simulink library "Ultrastick_Aero_Lib"  (Simulink 7.5)
settings: Solver=ode45  StartTime=0.0  StopTime=10.0  RelTol=1e-3
values from neighbouring files (symbols this model uses):
  AC = FASER_config    [UAV_config.m]    (also in UAV_modelconfig.mat = )
libraries: simulink x2
settings Model: Creator=austinmurch  LastModifiedBy=austinmurch

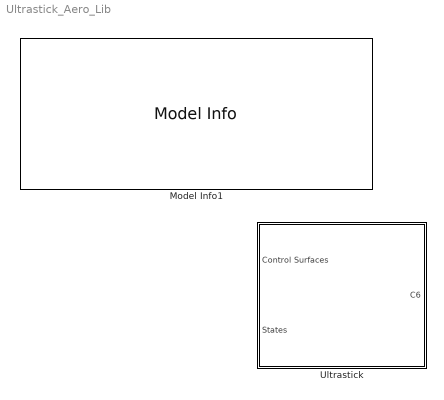
== system Ultrastick_Aero_Lib ==
  Model Info1 : simulink/Model-Wide Utilities/Model Info  SystemSampleTime=-1  InitialBlockCM=None  BlockCM=None  Frame=on  DisplayStringWithTags=|  HorizontalTextAlignment=Left  LeftAlignmentValue=0.02  SourceBlockDiagram=Ultrastick_Aero_Lib  TagMaxNumber=20
      | MODEL INFORMATION
      | Ultra Stick Aerodynamic Model Library
      | 
      | University of Minnesota
      | Aerospace Engineering and Mechanics
      | Copyright 2011 Regents of the University of Minnesota. All rights reserved.
      | 
      | == SVN Info ==
      | %<ModelVersion>
      | Last modified by %<LastModifiedBy> on %<LastModificationDate>
  Ultrastick : Subsystem

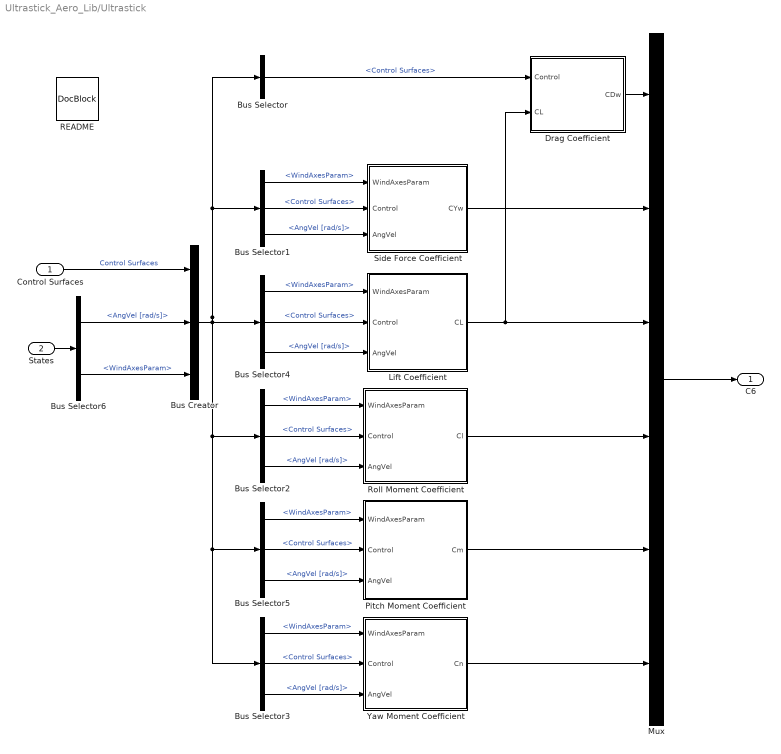
== system Ultrastick_Aero_Lib/Ultrastick ==
  Control Surfaces : Inport
  States : Inport  Port=2  OutDataType=sfix(16)  OutScaling=2^0
  Bus Creator : BusCreator  Inputs=3
  Bus Selector : BusSelector  OutputSignals=Control Surfaces
  Bus Selector{1..5} (5 alike) : BusSelector  OutputSignals=WindAxesParam,Control Surfaces,AngVel [rad/s]
  Bus Selector6 : BusSelector  OutputSignals=AngVel [rad/s],WindAxesParam
  Drag Coefficient : Subsystem
  Lift Coefficient : Subsystem
  Mux : Mux  Inputs=6
  Pitch Moment Coefficient : Subsystem
  README : simulink/Model-Wide Utilities/DocBlock  SystemSampleTime=-1  DocumentType=Text
  Roll Moment Coefficient : Subsystem
  Side Force Coefficient : Subsystem
  Yaw Moment Coefficient : Subsystem
  C6 : Outport  OutDataType=sfix(16)  OutScaling=2^0
  wires:
  Bus Selector/1 -> Drag Coefficient/1(Control)  "<Control Surfaces>"
  Control Surfaces/1 -> Bus Creator/1  "Control Surfaces"
  Bus Selector5/3 -> Pitch Moment Coefficient/3(AngVel)  "<AngVel [rad/s]>"
  Bus Selector5/2 -> Pitch Moment Coefficient/2(Control)  "<Control Surfaces>"
  Bus Selector5/1 -> Pitch Moment Coefficient/1(WindAxesParam)  "<WindAxesParam>"
  Bus Selector4/3 -> Lift Coefficient/3(AngVel)  "<AngVel [rad/s]>"
  Bus Selector4/2 -> Lift Coefficient/2(Control)  "<Control Surfaces>"
  Bus Selector4/1 -> Lift Coefficient/1(WindAxesParam)  "<WindAxesParam>"
  Bus Selector3/3 -> Yaw Moment Coefficient/3(AngVel)  "<AngVel [rad/s]>"
  Bus Selector3/2 -> Yaw Moment Coefficient/2(Control)  "<Control Surfaces>"
  Bus Selector3/1 -> Yaw Moment Coefficient/1(WindAxesParam)  "<WindAxesParam>"
  Bus Selector2/3 -> Roll Moment Coefficient/3(AngVel)  "<AngVel [rad/s]>"
  Bus Selector2/2 -> Roll Moment Coefficient/2(Control)  "<Control Surfaces>"
  Bus Selector2/1 -> Roll Moment Coefficient/1(WindAxesParam)  "<WindAxesParam>"
  Bus Selector1/3 -> Side Force Coefficient/3(AngVel)  "<AngVel [rad/s]>"
  Bus Selector1/2 -> Side Force Coefficient/2(Control)  "<Control Surfaces>"
  Bus Selector1/1 -> Side Force Coefficient/1(WindAxesParam)  "<WindAxesParam>"
  Bus Creator/1 -> Bus Selector4/1, Bus Selector1/1, Bus Selector/1, Bus Selector5/1, Bus Selector3/1, Bus Selector2/1
  Mux/1 -> C6/1
  Yaw Moment Coefficient/1(Cn) -> Mux/6
  Pitch Moment Coefficient/1(Cm) -> Mux/5
  Roll Moment Coefficient/1(Cl) -> Mux/4
  Side Force Coefficient/1(CYw) -> Mux/2
  Drag Coefficient/1(CDw) -> Mux/1
  States/1 -> Bus Selector6/1
  Bus Selector6/1 -> Bus Creator/2  "<AngVel [rad/s]>"
  Bus Selector6/2 -> Bus Creator/3  "<WindAxesParam>"
  Lift Coefficient/1(CL) -> Mux/3, Drag Coefficient/2(CL)

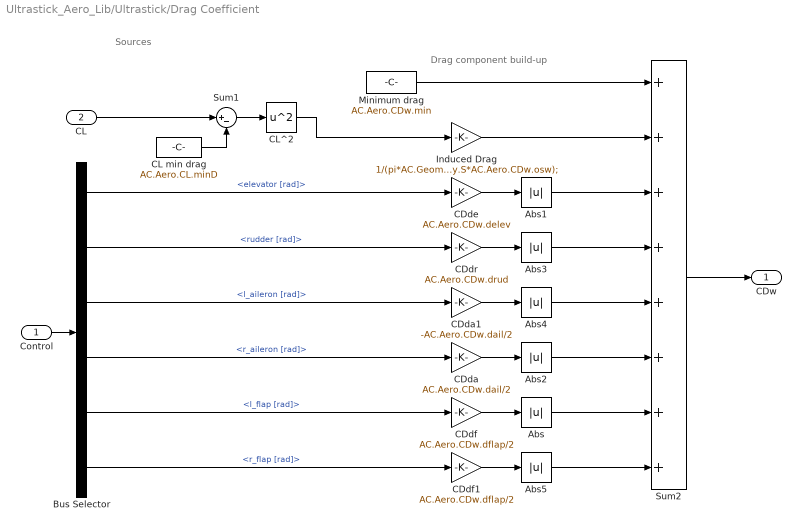
== system Ultrastick_Aero_Lib/Ultrastick/Drag Coefficient ==
  note: Drag component build-up
  note: Sources
  Control : Inport  OutDataType=sfix(16)  OutScaling=2^0
  CL : Inport  Port=2  OutDataType=sfix(16)  OutScaling=2^0
  Abs{,1..5} (6 alike) : Abs  SaturateOnIntegerOverflow=on
  Bus Selector : BusSelector  OutputSignals=elevator [rad],rudder [rad],l_aileron [rad],r_aileron [rad],l_flap [rad],r_flap [rad]
  CDda : Gain  Gain=AC.Aero.CDw.dail/2  ParameterDataType=sfix(16)  ParameterScaling=2^0  OutDataType=sfix(16)  OutScaling=2^0  SaturateOnIntegerOverflow=on  OutDataTypeStr=Inherit: Same as input  ParamDataTypeStr=Inherit: Same as input
  CDda1 : Gain  Gain=-AC.Aero.CDw.dail/2  ParameterDataType=sfix(16)  ParameterScaling=2^0  OutDataType=sfix(16)  OutScaling=2^0  SaturateOnIntegerOverflow=on  OutDataTypeStr=Inherit: Same as input  ParamDataTypeStr=Inherit: Same as input
  CDde : Gain  Gain=AC.Aero.CDw.delev  ParameterDataType=sfix(16)  ParameterScaling=2^0  OutDataType=sfix(16)  OutScaling=2^0  SaturateOnIntegerOverflow=on  OutDataTypeStr=Inherit: Same as input  ParamDataTypeStr=Inherit: Same as input
  CDdf : Gain  Gain=AC.Aero.CDw.dflap/2  ParameterDataType=sfix(16)  ParameterScaling=2^0  OutDataType=sfix(16)  OutScaling=2^0  SaturateOnIntegerOverflow=on  OutDataTypeStr=Inherit: Same as input  ParamDataTypeStr=Inherit: Same as input
  CDdf1 : Gain  Gain=AC.Aero.CDw.dflap/2  ParameterDataType=sfix(16)  ParameterScaling=2^0  OutDataType=sfix(16)  OutScaling=2^0  SaturateOnIntegerOverflow=on  OutDataTypeStr=Inherit: Same as input  ParamDataTypeStr=Inherit: Same as input
  CDdr : Gain  Gain=AC.Aero.CDw.drud  ParameterDataType=sfix(16)  ParameterScaling=2^0  OutDataType=sfix(16)  OutScaling=2^0  SaturateOnIntegerOverflow=on  OutDataTypeStr=Inherit: Same as input  ParamDataTypeStr=Inherit: Same as input
  CL min drag : Constant  Value=AC.Aero.CL.minD  OutDataType=sfix(16)  OutScaling=2^0
  CL^2 : Math  Operator=square  SaturateOnIntegerOverflow=on
  Induced Drag : Gain  Gain=1/(pi*AC.Geometry.b^2/AC.Geometry.S*AC.Aero.CDw.osw);  ParameterDataType=sfix(16)  ParameterScaling=2^0  OutDataType=sfix(16)  OutScaling=2^0  SaturateOnIntegerOverflow=on  OutDataTypeStr=Inherit: Same as input  ParamDataTypeStr=Inherit: Same as input
  Minimum drag : Constant  Value=AC.Aero.CDw.min  OutDataType=sfix(16)  OutScaling=2^0
  Sum1 : Sum  Inputs=|+-  OutDataType=sfix(16)  OutScaling=2^0  SaturateOnIntegerOverflow=on  InputSameDT=on  OutDataTypeStr=Inherit: Same as first input
  Sum2 : Sum  Inputs=++++++++  OutDataType=sfix(16)  OutScaling=2^0  SaturateOnIntegerOverflow=on  InputSameDT=on  OutDataTypeStr=Inherit: Same as first input
  CDw : Outport
  wires:
  Bus Selector/6 -> CDdf1/1  "<r_flap [rad]>"
  Abs/1 -> Sum2/7
  Abs5/1 -> Sum2/8
  CDdf1/1 -> Abs5/1
  Bus Selector/3 -> CDda1/1  "<l_aileron [rad]>"
  Abs4/1 -> Sum2/5
  CDda1/1 -> Abs4/1
  Abs2/1 -> Sum2/6
  Bus Selector/4 -> CDda/1  "<r_aileron [rad]>"
  Abs3/1 -> Sum2/4
  Abs1/1 -> Sum2/3
  CL min drag/1 -> Sum1/2
  CL/1 -> Sum1/1
  Sum1/1 -> CL^2/1
  Sum2/1 -> CDw/1
  CDdr/1 -> Abs3/1
  CDda/1 -> Abs2/1
  CDde/1 -> Abs1/1
  CDdf/1 -> Abs/1
  Induced Drag/1 -> Sum2/2
  Minimum drag/1 -> Sum2/1
  CL^2/1 -> Induced Drag/1
  Control/1 -> Bus Selector/1
  Bus Selector/2 -> CDdr/1  "<rudder [rad]>"
  Bus Selector/1 -> CDde/1  "<elevator [rad]>"
  Bus Selector/5 -> CDdf/1  "<l_flap [rad]>"

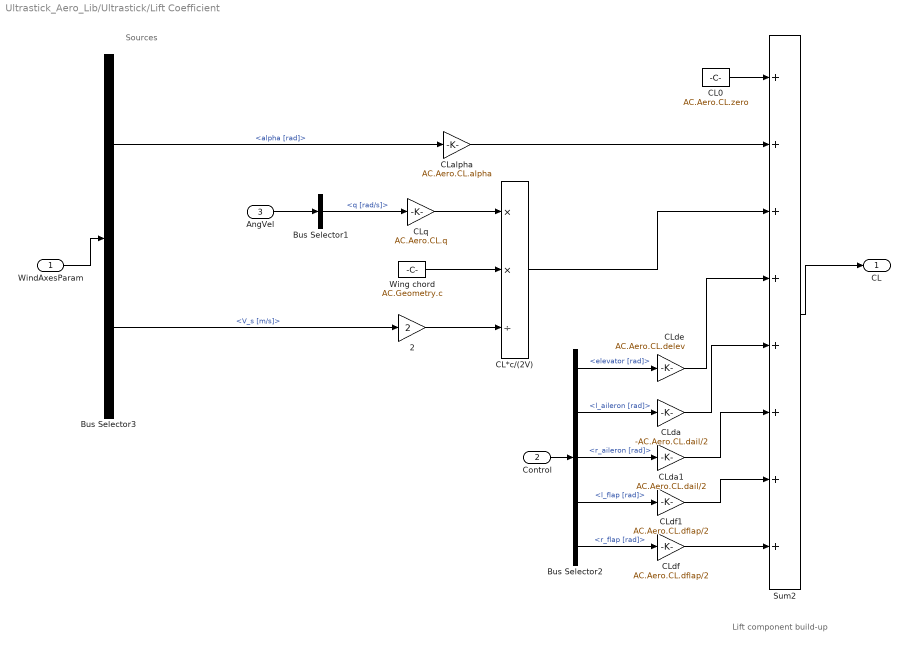
== system Ultrastick_Aero_Lib/Ultrastick/Lift Coefficient ==
  note: Lift component build-up
  note: Sources
  WindAxesParam : Inport  OutDataType=sfix(16)  OutScaling=2^0
  Control : Inport  Port=2  OutDataType=sfix(16)  OutScaling=2^0
  AngVel : Inport  Port=3  OutDataType=sfix(16)  OutScaling=2^0
  2 : Gain  Gain=2  ParameterDataType=sfix(16)  ParameterScaling=2^0  OutDataType=sfix(16)  OutScaling=2^0  SaturateOnIntegerOverflow=on  OutDataTypeStr=Inherit: Same as input  ParamDataTypeStr=Inherit: Same as input
  Bus Selector1 : BusSelector  OutputSignals=q [rad/s]
  Bus Selector2 : BusSelector  OutputSignals=elevator [rad],l_aileron [rad],r_aileron [rad],l_flap [rad],r_flap [rad]
  Bus Selector3 : BusSelector  OutputSignals=alpha [rad],V_s [m/s]
  CL*c/(2V) : Product  Inputs=**/  OutDataType=sfix(16)  OutScaling=2^0  SaturateOnIntegerOverflow=on  InputSameDT=on  OutDataTypeStr=Inherit: Same as first input
  CL0 : Constant  Value=AC.Aero.CL.zero  OutDataType=sfix(16)  OutScaling=2^0
  CLalpha : Gain  Gain=AC.Aero.CL.alpha  ParameterDataType=sfix(16)  ParameterScaling=2^0  OutDataType=sfix(16)  OutScaling=2^0  SaturateOnIntegerOverflow=on  OutDataTypeStr=Inherit: Same as input  ParamDataTypeStr=Inherit: Same as input
  CLda : Gain  Gain=-AC.Aero.CL.dail/2  ParameterDataType=sfix(16)  ParameterScaling=2^0  OutDataType=sfix(16)  OutScaling=2^0  SaturateOnIntegerOverflow=on  OutDataTypeStr=Inherit: Same as input  ParamDataTypeStr=Inherit: Same as input
  CLda1 : Gain  Gain=AC.Aero.CL.dail/2  ParameterDataType=sfix(16)  ParameterScaling=2^0  OutDataType=sfix(16)  OutScaling=2^0  SaturateOnIntegerOverflow=on  OutDataTypeStr=Inherit: Same as input  ParamDataTypeStr=Inherit: Same as input
  CLde : Gain  Gain=AC.Aero.CL.delev  ParameterDataType=sfix(16)  ParameterScaling=2^0  OutDataType=sfix(16)  OutScaling=2^0  SaturateOnIntegerOverflow=on  OutDataTypeStr=Inherit: Same as input  ParamDataTypeStr=Inherit: Same as input
  CLdf : Gain  Gain=AC.Aero.CL.dflap/2  ParameterDataType=sfix(16)  ParameterScaling=2^0  OutDataType=sfix(16)  OutScaling=2^0  SaturateOnIntegerOverflow=on  OutDataTypeStr=Inherit: Same as input  ParamDataTypeStr=Inherit: Same as input
  CLdf1 : Gain  Gain=AC.Aero.CL.dflap/2  ParameterDataType=sfix(16)  ParameterScaling=2^0  OutDataType=sfix(16)  OutScaling=2^0  SaturateOnIntegerOverflow=on  OutDataTypeStr=Inherit: Same as input  ParamDataTypeStr=Inherit: Same as input
  CLq : Gain  Gain=AC.Aero.CL.q  ParameterDataType=sfix(16)  ParameterScaling=2^0  OutDataType=sfix(16)  OutScaling=2^0  SaturateOnIntegerOverflow=on  OutDataTypeStr=Inherit: Same as input  ParamDataTypeStr=Inherit: Same as input
  Sum2 : Sum  Inputs=++++++++  OutDataType=sfix(16)  OutScaling=2^0  SaturateOnIntegerOverflow=on  InputSameDT=on  OutDataTypeStr=Inherit: Same as first input
  Wing chord : Constant  Value=AC.Geometry.c  OutDataType=sfix(16)  OutScaling=2^0
  CL : Outport
  wires:
  CLda/1 -> Sum2/5
  CLda1/1 -> Sum2/6
  CLdf/1 -> Sum2/8
  CLdf1/1 -> Sum2/7
  Bus Selector2/5 -> CLdf/1  "<r_flap [rad]>"
  Bus Selector2/4 -> CLdf1/1  "<l_flap [rad]>"
  Bus Selector2/3 -> CLda1/1  "<r_aileron [rad]>"
  Bus Selector2/2 -> CLda/1  "<l_aileron [rad]>"
  CLde/1 -> Sum2/4
  CL*c/(2V)/1 -> Sum2/3
  Bus Selector3/2 -> 2/1  "<V_s [m/s]>"
  Bus Selector1/1 -> CLq/1  "<q [rad/s]>"
  AngVel/1 -> Bus Selector1/1
  CLq/1 -> CL*c/(2V)/1
  Wing chord/1 -> CL*c/(2V)/2
  2/1 -> CL*c/(2V)/3
  Bus Selector2/1 -> CLde/1  "<elevator [rad]>"
  Control/1 -> Bus Selector2/1
  Bus Selector3/1 -> CLalpha/1  "<alpha [rad]>"
  Sum2/1 -> CL/1
  CLalpha/1 -> Sum2/2
  CL0/1 -> Sum2/1
  WindAxesParam/1 -> Bus Selector3/1

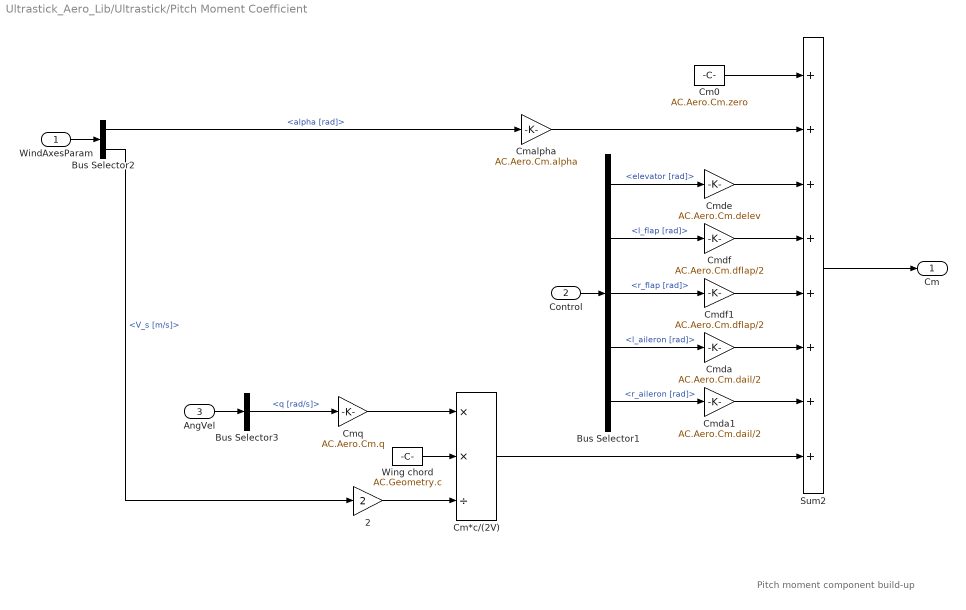
== system Ultrastick_Aero_Lib/Ultrastick/Pitch Moment Coefficient ==
  note: Pitch moment component build-up
  WindAxesParam : Inport
  Control : Inport  Port=2
  AngVel : Inport  Port=3
  2 : Gain  Gain=2  SaturateOnIntegerOverflow=on  OutDataTypeStr=Inherit: Same as input  ParamDataTypeStr=Inherit: Same as input
  Bus Selector1 : BusSelector  OutputSignals=elevator [rad],l_flap [rad],r_flap [rad],l_aileron [rad],r_aileron [rad]
  Bus Selector2 : BusSelector  OutputSignals=alpha [rad],V_s [m/s]
  Bus Selector3 : BusSelector  OutputSignals=q [rad/s]
  Cm*c/(2V) : Product  Inputs=**/  SaturateOnIntegerOverflow=on  RndMeth=Zero  InputSameDT=on  OutDataTypeStr=Inherit: Same as first input
  Cm0 : Constant  Value=AC.Aero.Cm.zero
  Cmalpha : Gain  Gain=AC.Aero.Cm.alpha  SaturateOnIntegerOverflow=on  OutDataTypeStr=Inherit: Same as input  ParamDataTypeStr=Inherit: Same as input
  Cmda : Gain  Gain=AC.Aero.Cm.dail/2  SaturateOnIntegerOverflow=on  OutDataTypeStr=Inherit: Same as input  ParamDataTypeStr=Inherit: Same as input
  Cmda1 : Gain  Gain=AC.Aero.Cm.dail/2  SaturateOnIntegerOverflow=on  OutDataTypeStr=Inherit: Same as input  ParamDataTypeStr=Inherit: Same as input
  Cmde : Gain  Gain=AC.Aero.Cm.delev  SaturateOnIntegerOverflow=on  OutDataTypeStr=Inherit: Same as input  ParamDataTypeStr=Inherit: Same as input
  Cmdf : Gain  Gain=AC.Aero.Cm.dflap/2  SaturateOnIntegerOverflow=on  OutDataTypeStr=Inherit: Same as input  ParamDataTypeStr=Inherit: Same as input
  Cmdf1 : Gain  Gain=AC.Aero.Cm.dflap/2  SaturateOnIntegerOverflow=on  OutDataTypeStr=Inherit: Same as input  ParamDataTypeStr=Inherit: Same as input
  Cmq : Gain  Gain=AC.Aero.Cm.q  SaturateOnIntegerOverflow=on  OutDataTypeStr=Inherit: Same as input  ParamDataTypeStr=Inherit: Same as input
  Sum2 : Sum  Inputs=++++++++  SaturateOnIntegerOverflow=on  InputSameDT=on  OutDataTypeStr=Inherit: Same as first input
  Wing chord : Constant  Value=AC.Geometry.c
  Cm : Outport
  wires:
  Bus Selector1/5 -> Cmda1/1  "<r_aileron [rad]>"
  Bus Selector1/4 -> Cmda/1  "<l_aileron [rad]>"
  Bus Selector1/3 -> Cmdf1/1  "<r_flap [rad]>"
  Bus Selector1/2 -> Cmdf/1  "<l_flap [rad]>"
  Bus Selector1/1 -> Cmde/1  "<elevator [rad]>"
  Cmda1/1 -> Sum2/7
  Cmda/1 -> Sum2/6
  Cmdf1/1 -> Sum2/5
  Cmdf/1 -> Sum2/4
  Cmde/1 -> Sum2/3
  Cm*c/(2V)/1 -> Sum2/8
  Bus Selector2/2 -> 2/1  "<V_s [m/s]>"
  Bus Selector2/1 -> Cmalpha/1  "<alpha [rad]>"
  Bus Selector3/1 -> Cmq/1  "<q [rad/s]>"
  Sum2/1 -> Cm/1
  Cmalpha/1 -> Sum2/2
  Cm0/1 -> Sum2/1
  Cmq/1 -> Cm*c/(2V)/1
  Wing chord/1 -> Cm*c/(2V)/2
  2/1 -> Cm*c/(2V)/3
  AngVel/1 -> Bus Selector3/1
  Control/1 -> Bus Selector1/1
  WindAxesParam/1 -> Bus Selector2/1

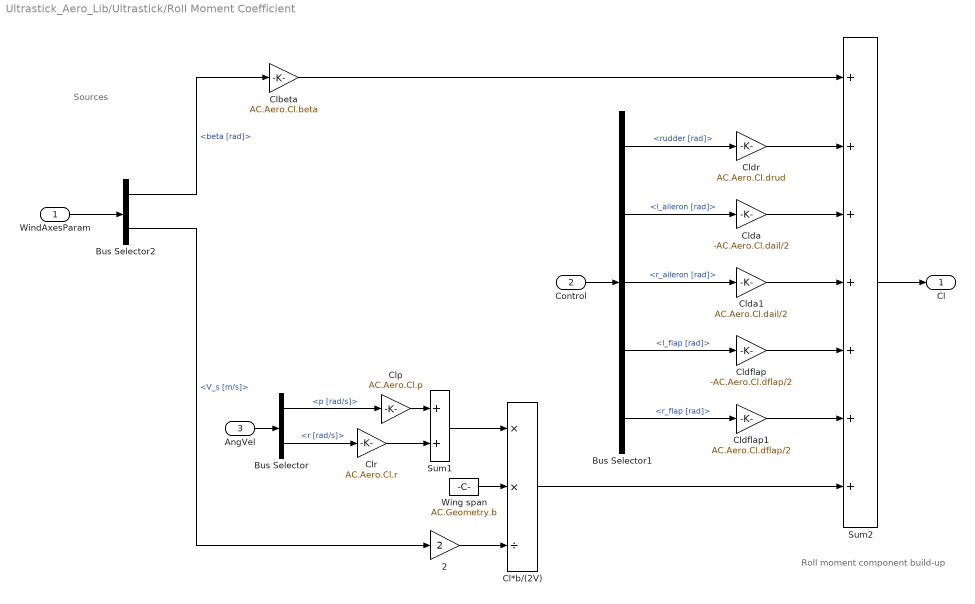
== system Ultrastick_Aero_Lib/Ultrastick/Roll Moment Coefficient ==
  note: Roll moment component build-up
  note: Sources
  WindAxesParam : Inport
  Control : Inport  Port=2
  AngVel : Inport  Port=3
  2 : Gain  Gain=2  SaturateOnIntegerOverflow=on  OutDataTypeStr=Inherit: Same as input  ParamDataTypeStr=Inherit: Same as input
  Bus Selector : BusSelector  OutputSignals=p [rad/s],r [rad/s]
  Bus Selector1 : BusSelector  OutputSignals=rudder [rad],l_aileron [rad],r_aileron [rad],l_flap [rad],r_flap [rad]
  Bus Selector2 : BusSelector  OutputSignals=beta [rad],V_s [m/s]
  Cl*b/(2V) : Product  Inputs=**/  SaturateOnIntegerOverflow=on  RndMeth=Zero  InputSameDT=on  OutDataTypeStr=Inherit: Same as first input
  Clbeta : Gain  Gain=AC.Aero.Cl.beta  SaturateOnIntegerOverflow=on  OutDataTypeStr=Inherit: Same as input  ParamDataTypeStr=Inherit: Same as input
  Clda : Gain  Gain=-AC.Aero.Cl.dail/2  SaturateOnIntegerOverflow=on  OutDataTypeStr=Inherit: Same as input  ParamDataTypeStr=Inherit: Same as input
  Clda1 : Gain  Gain=AC.Aero.Cl.dail/2  SaturateOnIntegerOverflow=on  OutDataTypeStr=Inherit: Same as input  ParamDataTypeStr=Inherit: Same as input
  Cldflap : Gain  Gain=-AC.Aero.Cl.dflap/2  SaturateOnIntegerOverflow=on  OutDataTypeStr=Inherit: Same as input  ParamDataTypeStr=Inherit: Same as input
  Cldflap1 : Gain  Gain=AC.Aero.Cl.dflap/2  SaturateOnIntegerOverflow=on  OutDataTypeStr=Inherit: Same as input  ParamDataTypeStr=Inherit: Same as input
  Cldr : Gain  Gain=AC.Aero.Cl.drud  SaturateOnIntegerOverflow=on  OutDataTypeStr=Inherit: Same as input  ParamDataTypeStr=Inherit: Same as input
  Clp : Gain  Gain=AC.Aero.Cl.p  SaturateOnIntegerOverflow=on  OutDataTypeStr=Inherit: Same as input  ParamDataTypeStr=Inherit: Same as input
  Clr : Gain  Gain=AC.Aero.Cl.r  SaturateOnIntegerOverflow=on  OutDataTypeStr=Inherit: Same as input  ParamDataTypeStr=Inherit: Same as input
  Sum1 : Sum  SaturateOnIntegerOverflow=on  InputSameDT=on  OutDataTypeStr=Inherit: Same as first input
  Sum2 : Sum  Inputs=+++++++  SaturateOnIntegerOverflow=on  InputSameDT=on  OutDataTypeStr=Inherit: Same as first input
  Wing span : Constant  Value=AC.Geometry.b
  Cl : Outport
  wires:
  Cldflap1/1 -> Sum2/6
  Cldflap/1 -> Sum2/5
  Bus Selector1/5 -> Cldflap1/1  "<r_flap [rad]>"
  Bus Selector1/4 -> Cldflap/1  "<l_flap [rad]>"
  Clda1/1 -> Sum2/4
  Bus Selector1/3 -> Clda1/1  "<r_aileron [rad]>"
  Bus Selector1/2 -> Clda/1  "<l_aileron [rad]>"
  Clda/1 -> Sum2/3
  Cl*b/(2V)/1 -> Sum2/7
  Cldr/1 -> Sum2/2
  Bus Selector2/2 -> 2/1  "<V_s [m/s]>"
  Bus Selector2/1 -> Clbeta/1  "<beta [rad]>"
  Bus Selector1/1 -> Cldr/1  "<rudder [rad]>"
  Control/1 -> Bus Selector1/1
  Bus Selector/2 -> Clr/1  "<r [rad/s]>"
  Bus Selector/1 -> Clp/1  "<p [rad/s]>"
  Sum2/1 -> Cl/1
  Clbeta/1 -> Sum2/1
  AngVel/1 -> Bus Selector/1
  WindAxesParam/1 -> Bus Selector2/1
  2/1 -> Cl*b/(2V)/3
  Wing span/1 -> Cl*b/(2V)/2
  Sum1/1 -> Cl*b/(2V)/1
  Clr/1 -> Sum1/2
  Clp/1 -> Sum1/1

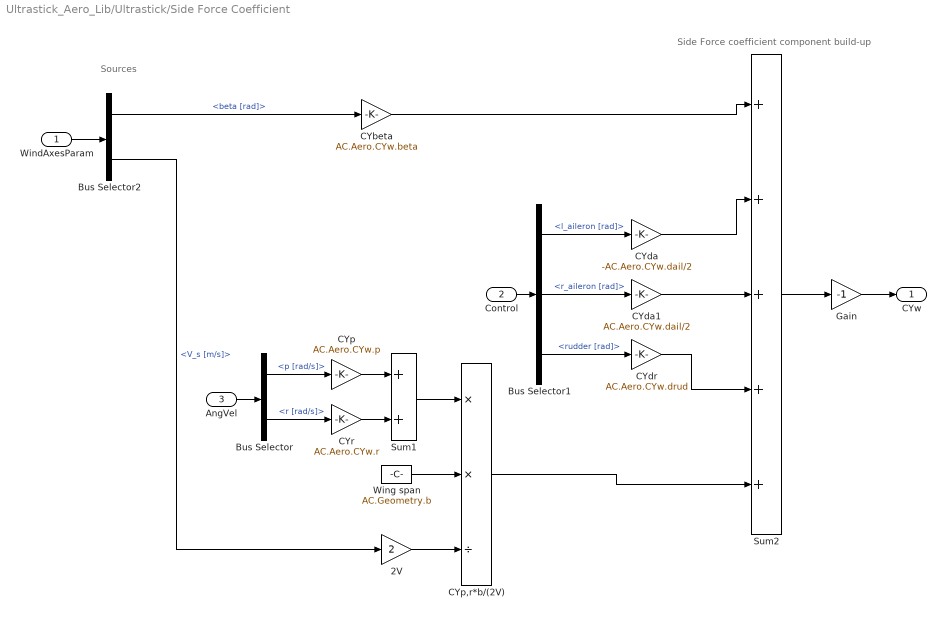
== system Ultrastick_Aero_Lib/Ultrastick/Side Force Coefficient ==
  note: Side Force coefficient component build-up
  note: Sources
  WindAxesParam : Inport
  Control : Inport  Port=2
  AngVel : Inport  Port=3
  2V : Gain  Gain=2  SaturateOnIntegerOverflow=on  OutDataTypeStr=Inherit: Same as input  ParamDataTypeStr=Inherit: Same as input
  Bus Selector : BusSelector  OutputSignals=p [rad/s],r [rad/s]
  Bus Selector1 : BusSelector  OutputSignals=l_aileron [rad],r_aileron [rad],rudder [rad]
  Bus Selector2 : BusSelector  OutputSignals=beta [rad],V_s [m/s]
  CYbeta : Gain  Gain=AC.Aero.CYw.beta  SaturateOnIntegerOverflow=on  OutDataTypeStr=Inherit: Same as input  ParamDataTypeStr=Inherit: Same as input
  CYda : Gain  Gain=-AC.Aero.CYw.dail/2  SaturateOnIntegerOverflow=on  OutDataTypeStr=Inherit: Same as input  ParamDataTypeStr=Inherit: Same as input
  CYda1 : Gain  Gain=AC.Aero.CYw.dail/2  SaturateOnIntegerOverflow=on  OutDataTypeStr=Inherit: Same as input  ParamDataTypeStr=Inherit: Same as input
  CYdr : Gain  Gain=AC.Aero.CYw.drud  SaturateOnIntegerOverflow=on  OutDataTypeStr=Inherit: Same as input  ParamDataTypeStr=Inherit: Same as input
  CYp : Gain  Gain=AC.Aero.CYw.p  SaturateOnIntegerOverflow=on  OutDataTypeStr=Inherit: Same as input  ParamDataTypeStr=Inherit: Same as input
  CYp,r*b/(2V) : Product  Inputs=**/  SaturateOnIntegerOverflow=on  RndMeth=Zero  InputSameDT=on  OutDataTypeStr=Inherit: Same as first input
  CYr : Gain  Gain=AC.Aero.CYw.r  SaturateOnIntegerOverflow=on  OutDataTypeStr=Inherit: Same as input  ParamDataTypeStr=Inherit: Same as input
  Gain : Gain  Gain=-1  ParameterDataType=fixdt(1, 16)  ParameterScaling=2^0  OutDataType=fixdt(1, 16)  OutScaling=2^0
  Sum1 : Sum  SaturateOnIntegerOverflow=on  InputSameDT=on  OutDataTypeStr=Inherit: Same as first input
  Sum2 : Sum  Inputs=+++++  SaturateOnIntegerOverflow=on  InputSameDT=on  OutDataTypeStr=Inherit: Same as first input
  Wing span : Constant  Value=AC.Geometry.b
  CYw : Outport
  wires:
  CYda1/1 -> Sum2/3
  Bus Selector1/2 -> CYda1/1  "<r_aileron [rad]>"
  CYdr/1 -> Sum2/4
  CYp,r*b/(2V)/1 -> Sum2/5
  Gain/1 -> CYw/1
  Bus Selector2/1 -> CYbeta/1  "<beta [rad]>"
  Bus Selector2/2 -> 2V/1  "<V_s [m/s]>"
  Bus Selector1/3 -> CYdr/1  "<rudder [rad]>"
  Bus Selector1/1 -> CYda/1  "<l_aileron [rad]>"
  Control/1 -> Bus Selector1/1
  Bus Selector/2 -> CYr/1  "<r [rad/s]>"
  AngVel/1 -> Bus Selector/1
  Sum2/1 -> Gain/1
  CYda/1 -> Sum2/2
  CYbeta/1 -> Sum2/1
  Bus Selector/1 -> CYp/1  "<p [rad/s]>"
  WindAxesParam/1 -> Bus Selector2/1
  2V/1 -> CYp,r*b/(2V)/3
  Wing span/1 -> CYp,r*b/(2V)/2
  Sum1/1 -> CYp,r*b/(2V)/1
  CYr/1 -> Sum1/2
  CYp/1 -> Sum1/1

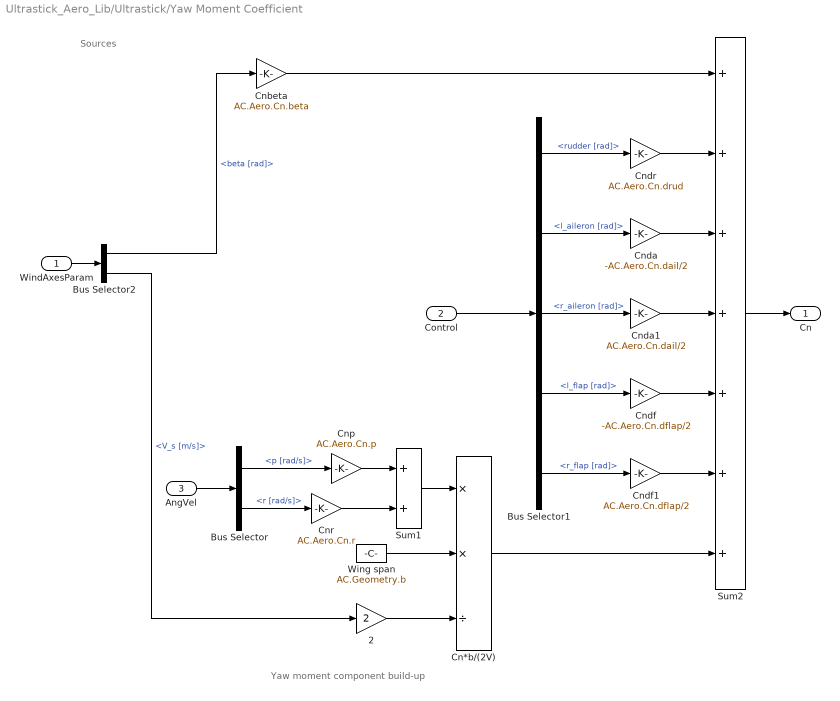
== system Ultrastick_Aero_Lib/Ultrastick/Yaw Moment Coefficient ==
  note: Sources
  note: Yaw moment component build-up
  WindAxesParam : Inport
  Control : Inport  Port=2
  AngVel : Inport  Port=3
  2 : Gain  Gain=2  SaturateOnIntegerOverflow=on  OutDataTypeStr=Inherit: Same as input  ParamDataTypeStr=Inherit: Same as input
  Bus Selector : BusSelector  OutputSignals=p [rad/s],r [rad/s]
  Bus Selector1 : BusSelector  OutputSignals=rudder [rad],l_aileron [rad],r_aileron [rad],l_flap [rad],r_flap [rad]
  Bus Selector2 : BusSelector  OutputSignals=beta [rad],V_s [m/s]
  Cn*b/(2V) : Product  Inputs=**/  SaturateOnIntegerOverflow=on  RndMeth=Zero  InputSameDT=on  OutDataTypeStr=Inherit: Same as first input
  Cnbeta : Gain  Gain=AC.Aero.Cn.beta  SaturateOnIntegerOverflow=on  OutDataTypeStr=Inherit: Same as input  ParamDataTypeStr=Inherit: Same as input
  Cnda : Gain  Gain=-AC.Aero.Cn.dail/2  SaturateOnIntegerOverflow=on  OutDataTypeStr=Inherit: Same as input  ParamDataTypeStr=Inherit: Same as input
  Cnda1 : Gain  Gain=AC.Aero.Cn.dail/2  SaturateOnIntegerOverflow=on  OutDataTypeStr=Inherit: Same as input  ParamDataTypeStr=Inherit: Same as input
  Cndf : Gain  Gain=-AC.Aero.Cn.dflap/2  SaturateOnIntegerOverflow=on  OutDataTypeStr=Inherit: Same as input  ParamDataTypeStr=Inherit: Same as input
  Cndf1 : Gain  Gain=AC.Aero.Cn.dflap/2  SaturateOnIntegerOverflow=on  OutDataTypeStr=Inherit: Same as input  ParamDataTypeStr=Inherit: Same as input
  Cndr : Gain  Gain=AC.Aero.Cn.drud  SaturateOnIntegerOverflow=on  OutDataTypeStr=Inherit: Same as input  ParamDataTypeStr=Inherit: Same as input
  Cnp : Gain  Gain=AC.Aero.Cn.p  SaturateOnIntegerOverflow=on  OutDataTypeStr=Inherit: Same as input  ParamDataTypeStr=Inherit: Same as input
  Cnr : Gain  Gain=AC.Aero.Cn.r  SaturateOnIntegerOverflow=on  OutDataTypeStr=Inherit: Same as input  ParamDataTypeStr=Inherit: Same as input
  Sum1 : Sum  SaturateOnIntegerOverflow=on  InputSameDT=on  OutDataTypeStr=Inherit: Same as first input
  Sum2 : Sum  Inputs=+++++++  SaturateOnIntegerOverflow=on  InputSameDT=on  OutDataTypeStr=Inherit: Same as first input
  Wing span : Constant  Value=AC.Geometry.b
  Cn : Outport
  wires:
  Cnda/1 -> Sum2/3
  Cndr/1 -> Sum2/2
  Bus Selector1/5 -> Cndf1/1  "<r_flap [rad]>"
  Bus Selector1/4 -> Cndf/1  "<l_flap [rad]>"
  Bus Selector1/3 -> Cnda1/1  "<r_aileron [rad]>"
  Bus Selector1/2 -> Cnda/1  "<l_aileron [rad]>"
  Bus Selector1/1 -> Cndr/1  "<rudder [rad]>"
  Cndf1/1 -> Sum2/6
  Cndf/1 -> Sum2/5
  Cnda1/1 -> Sum2/4
  Cn*b/(2V)/1 -> Sum2/7
  Bus Selector2/2 -> 2/1  "<V_s [m/s]>"
  Bus Selector2/1 -> Cnbeta/1  "<beta [rad]>"
  Control/1 -> Bus Selector1/1
  Bus Selector/2 -> Cnr/1  "<r [rad/s]>"
  Bus Selector/1 -> Cnp/1  "<p [rad/s]>"
  Cnp/1 -> Sum1/1
  Cnr/1 -> Sum1/2
  Sum1/1 -> Cn*b/(2V)/1
  Wing span/1 -> Cn*b/(2V)/2
  2/1 -> Cn*b/(2V)/3
  WindAxesParam/1 -> Bus Selector2/1
  AngVel/1 -> Bus Selector/1
  Cnbeta/1 -> Sum2/1
  Sum2/1 -> Cn/1
